simulink model "perfect_differentiating"  (R2016a)
settings: Solver=VariableStepAuto  StartTime=0.0  StopTime=0.5  RelTol=1e-3
settings Model: Creator=Jann dan Jursus  LastModifiedBy=Jann dan Jursus

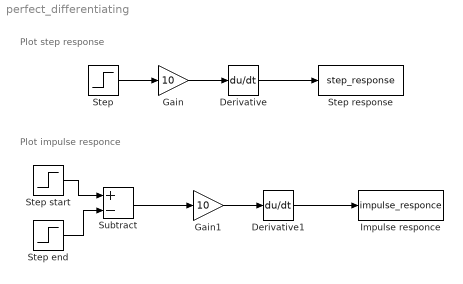
== system perfect_differentiating ==
  note: Plot impulse responce
  note: Plot step response
  Derivative : Derivative
  Derivative1 : Derivative
  Gain : Gain  Gain=10
  Gain1 : Gain  Gain=10
  Impulse responce : ToWorkspace  VariableName=impulse_responce  SaveFormat=Timeseries  SampleTime=-1
  Step : Step  Time=0  SampleTime=0
  Step end : Step  Time=1.001  After=100  SampleTime=0
  Step response : ToWorkspace  VariableName=step_response  SaveFormat=Timeseries  SampleTime=-1
  Step start : Step  After=100  SampleTime=0
  Subtract : Sum  Inputs=+-
  wires:
  Step start/1 -> Subtract/1
  Step end/1 -> Subtract/2
  Subtract/1 -> Gain1/1
  Step/1 -> Gain/1
  Gain/1 -> Derivative/1
  Derivative/1 -> Step response/1
  Gain1/1 -> Derivative1/1
  Derivative1/1 -> Impulse responce/1
